simulink model "exampleVapourContent"  (Simulink 7.6)
settings: Solver=ode45  StartTime=0.0  StopTime=10.0  RelTol=1e-3
libraries: carnot x3
settings Model: Creator=drhf  LastModifiedBy=drhf

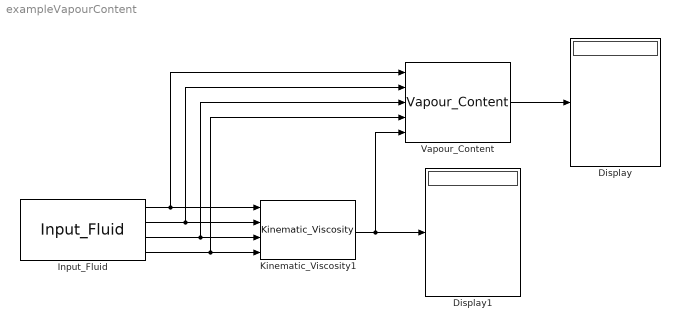
== system exampleVapourContent ==
  Display : Display
  Display1 : Display
  Input_Fluid : carnot/Basic/Material_Properties/Input_Fluid  SystemSampleTime=-1  fluid=water  T=[100:10:150]  p=1e5  x=0.005
  Kinematic_Viscosity1 : carnot/Basic/Material_Properties/Kinematic_Viscosity  SystemSampleTime=-1
  Vapour_Content : carnot/Basic/Material_Properties/Vapour_Content  SystemSampleTime=-1  prop=kinematic viscosity
  wires:
  Vapour_Content/1 -> Display/1
  Input_Fluid/1 -> Kinematic_Viscosity1/1, Vapour_Content/1
  Input_Fluid/2 -> Kinematic_Viscosity1/2, Vapour_Content/2
  Input_Fluid/3 -> Kinematic_Viscosity1/3, Vapour_Content/3
  Input_Fluid/4 -> Kinematic_Viscosity1/4, Vapour_Content/4
  Kinematic_Viscosity1/1 -> Display1/1, Vapour_Content/5
